simulink model "StopWatchHamon"  (Simulink 8.7)
settings: Solver=FixedStepDiscrete  StartTime=0.0  StopTime=100000.0  RelTol=1e-3
settings Model: Creator=scaife  LastModifiedBy=bourbouh  ExtModeAutoUpdateStatusClock=off
settings DataIOCC: SignalLoggingSaveFormat=ModelDataLogs  SignalLoggingName=sigsOut
settings DebuggingCC: SaveWithParameterizedLinksMsg=none  SignalResolutionControl=TryResolveAllWithWarning  MultiTaskDSMMsg=warning  MultiTaskCondExecSysMsg=none
settings HardwareCC: TargetUnknown=on
settings SFSimCC: SimParseCustomCode=off
settings GRTTargetCC: GeneratePreprocessorConditionals=Use local settings  CombineOutputUpdateFcns=off  GRTInterface=on

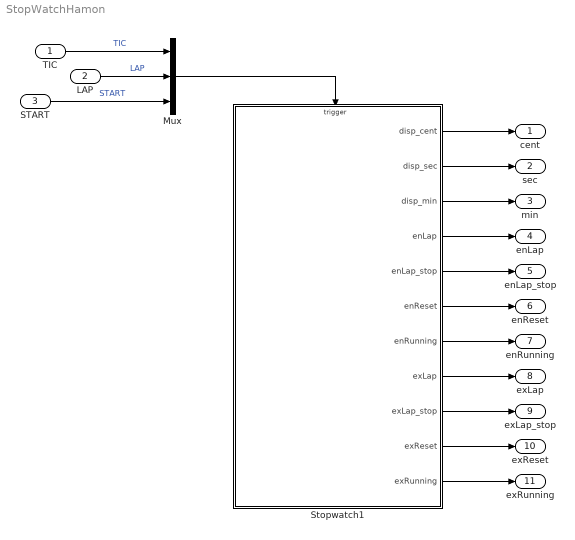
== system StopWatchHamon ==
  TIC : Inport
  LAP : Inport  Port=2
  START : Inport  Port=3
  Mux : Mux  Inputs=3
  Stopwatch1 : Stateflow chart  TreatAsAtomicUnit=on
  cent : Outport
  sec : Outport  Port=2
  min : Outport  Port=3
  enLap : Outport  Port=4
  enLap_stop : Outport  Port=5
  enReset : Outport  Port=6
  enRunning : Outport  Port=7
  exLap : Outport  Port=8
  exLap_stop : Outport  Port=9
  exReset : Outport  Port=10
  exRunning : Outport  Port=11
  wires:
  Stopwatch1/1(disp_cent) -> cent/1
  Stopwatch1/2(disp_sec) -> sec/1
  Stopwatch1/3(disp_min) -> min/1
  TIC/1 -> Mux/1  "TIC"
  LAP/1 -> Mux/2  "LAP"
  Mux/1 -> Stopwatch1/Trigger
  START/1 -> Mux/3  "START"
  Stopwatch1/4(enLap) -> enLap/1
  Stopwatch1/5(enLap_stop) -> enLap_stop/1
  Stopwatch1/6(enReset) -> enReset/1
  Stopwatch1/7(enRunning) -> enRunning/1
  Stopwatch1/8(exLap) -> exLap/1
  Stopwatch1/9(exLap_stop) -> exLap_stop/1
  Stopwatch1/10(exReset) -> exReset/1
  Stopwatch1/11(exRunning) -> exRunning/1

== stateflow chart Stopwatch1 ==
  state Stopwatch
    state Stop
      state Reset/
        en:
        enReset++;
        ex:
        exReset++;
        Reset -> (junction 10) [order 1] : LAP{ cent=0;
            | sec=0; min=0;
            | disp_cent=0;
            | disp_sec=0;
            | disp_min=0}
      state Lap_stop/
        en:
        enLap_stop++;
        ex:
        exLap_stop++;
      (default) -> Reset
      Lap_stop -> Reset [order 2] : LAP
    state Run
      state Lap/
        en:
        enLap++;
        ex:
        exLap++;
      state Running/
        en:
        enRunning++;
        during:
        disp_cent=cent;
        disp_sec=sec;
        disp_min=min;
        ex:
        exRunning++;
      Run -> (junction 19) : TIC{cent++;}
      (junction 19) -> (junction 21) [order 2]
      (junction 19) -> (junction 20) [order 1] : [cent==100]{cent=0; sec++;}
      Running -> Lap [order 2] : LAP
      Lap -> Running [order 2] : LAP
      (junction 20) -> (junction 21) [order 2]
      (junction 20) -> (junction 21) [order 1] : [sec==60]{sec=0; min++;}
    (default) -> Stop
    Reset -> Running [order 1] : START
    Running -> Reset [order 1] : START
    Lap_stop -> Lap [order 1] : START
    Lap -> Lap_stop [order 1] : START
  (default) -> Stopwatch
  data: cent local int32; sec local int32; min local int32; disp_cent output int32; disp_sec output int32; disp_min output int32; enLap output int32; enLap_stop output int32; enReset output int32; enRunning output int32; exLap output int32; exLap_stop output int32; exReset output int32; exRunning output int32
  events: TIC input EITHER_EDGE_EVENT; LAP input EITHER_EDGE_EVENT; START input EITHER_EDGE_EVENT
